simulink model "vipbarcoderecognition"  (R2015b)
settings: Solver=FixedStepDiscrete  StartTime=0.0  StopTime=inf  RelTol=1e-3
undefined symbols (not defined in the file or in its folder): gray, Rec, SDTV
libraries: visiontextngfix x2, simulink x1, visionconversions x1, visionsinks x1, dspvision x1, vipmisc x1
settings Model: FPTRunName=Active  Creator=The MathWorks, Inc.  LastModifiedBy=The MathWorks, Inc.
settings DataIOCC: SaveFormat=Array
settings OptimizationCC: ExpressionDepthLimit=2147483647  EfficientMapNaN2IntZero=off
settings DebuggingCC: UnderspecifiedInitializationDetection=Classic  MergeDetectMultiDrivingBlocksExec=none  SolverPrmCheckMsg=warning  FcnCallInpInsideContextMsg=UseLocalSettings  StateNameClashWarn=warning  StrictBusMsg=Warning
settings HardwareCC: ProdBitPerPointer=32  ProdLargestAtomicFloat=None  ProdIntDivRoundTo=Undefined  ProdEndianess=Unspecified  ProdWordSize=32  ProdHWDeviceType=32-bit Generic  TargetBitPerLong=64  TargetBitPerPointer=64  TargetLongLongMode=on  TargetIntDivRoundTo=Zero  TargetEndianess=LittleEndian  TargetWordSize=64  TargetHWDeviceType=Generic->MATLAB Host Computer  ProdEqTarget=off
settings SFSimCC: SimParseCustomCode=off
settings GRTTargetCC: GeneratePreprocessorConditionals=Disable all  CombineOutputUpdateFcns=off  GRTInterface=on
settings ConfigComp: CovModelRefEnable=Off

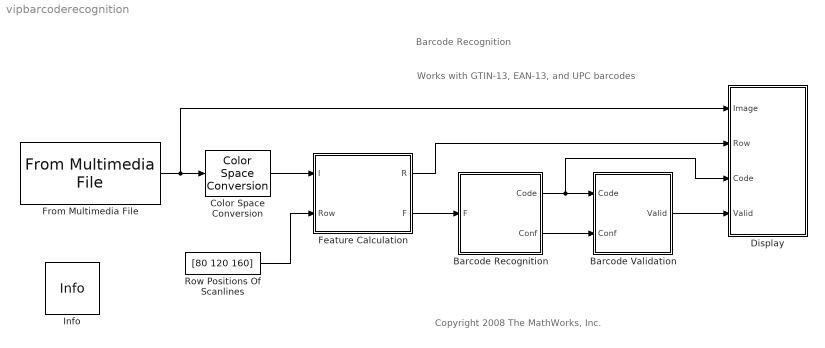
== system vipbarcoderecognition ==
  note: Barcode Recognition
  note: Copyright 2008 The MathWorks, Inc.
  note: Works with GTIN-13, EAN-13, and UPC barcodes
  Barcode Recognition : Subsystem
  Barcode Validation : Subsystem
  Color Space Conversion : visionconversions/Color Space  Conversion  conversion=Obsolete  conversionActive=R'G'B' to intensity  wp_str=D65  rec=Rec. 601 (SDTV)  sys=1125/60/2:1  imagePorts=One multidimensional signal
  Display : Subsystem
  Feature Calculation : MATLAB Function  TreatAsAtomicUnit=on
  From Multimedia File : dspvision/From Multimedia File  inputFilename=vipbarcode.avi  loop=on  numPlays=inf  outputStreams=Video only  videoDataType=single  audioDataType=int16  inheritSampleTime=on  userDefinedSampleTime=1/30  noAudioOutput=off  isIntensityVideo=off  fourcc=RGB  colorVideoFormat=One multidimensional signal  outputEOF=off  dataOrg=Column-major  audioFrameSize=1024  computeAudioFrameSize=off  outSamplingMode=Frame based
  Info : vipmisc/Info  SystemSampleTime=-1
  Row Positions Of Scanlines : Constant  Value=[80 120 160]  VectorParams1D=off  OutDataTypeStr=double
  wires:
  Color Space Conversion/1 -> Feature Calculation/1(I)
  Row Positions Of Scanlines/1 -> Feature Calculation/2(Row)
  From Multimedia File/1 -> Color Space Conversion/1, Display/1(Image)
  Feature Calculation/2(F) -> Barcode Recognition/1(F)
  Barcode Recognition/2(Conf) -> Barcode Validation/2(Conf)
  Barcode Recognition/1(Code) -> Barcode Validation/1(Code), Display/3(Code)
  Barcode Validation/1(Valid) -> Display/4(Valid)
  Feature Calculation/1(R) -> Display/2(Row)

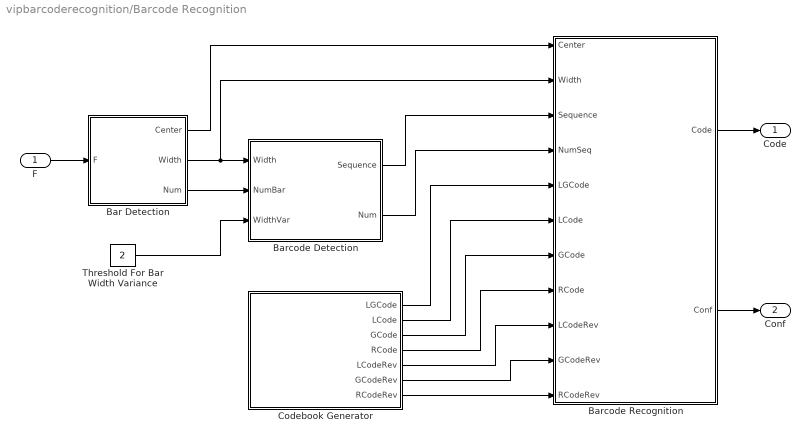
== system vipbarcoderecognition/Barcode Recognition ==
  F : Inport
  Bar Detection : MATLAB Function  TreatAsAtomicUnit=on
  Barcode Detection : MATLAB Function  TreatAsAtomicUnit=on
  Barcode Recognition : MATLAB Function  TreatAsAtomicUnit=on
  Codebook Generator : MATLAB Function  TreatAsAtomicUnit=on
  Threshold For Bar Width Variance : Constant  Value=2  VectorParams1D=off  OutDataTypeStr=single
  Code : Outport
  Conf : Outport  Port=2
  wires:
  Bar Detection/1(Center) -> Barcode Recognition/1(Center)
  Bar Detection/2(Width) -> Barcode Detection/1(Width), Barcode Recognition/2(Width)
  Bar Detection/3(Num) -> Barcode Detection/2(NumBar)
  Barcode Detection/1(Sequence) -> Barcode Recognition/3(Sequence)
  Barcode Detection/2(Num) -> Barcode Recognition/4(NumSeq)
  Codebook Generator/1(LGCode) -> Barcode Recognition/5(LGCode)
  Codebook Generator/2(LCode) -> Barcode Recognition/6(LCode)
  Codebook Generator/3(GCode) -> Barcode Recognition/7(GCode)
  Codebook Generator/4(RCode) -> Barcode Recognition/8(RCode)
  Codebook Generator/7(RCodeRev) -> Barcode Recognition/11(RCodeRev)
  Codebook Generator/5(LCodeRev) -> Barcode Recognition/9(LCodeRev)
  Codebook Generator/6(GCodeRev) -> Barcode Recognition/10(GCodeRev)
  Threshold For Bar Width Variance/1 -> Barcode Detection/3(WidthVar)
  Barcode Recognition/1(Code) -> Code/1
  F/1 -> Bar Detection/1(F)
  Barcode Recognition/2(Conf) -> Conf/1

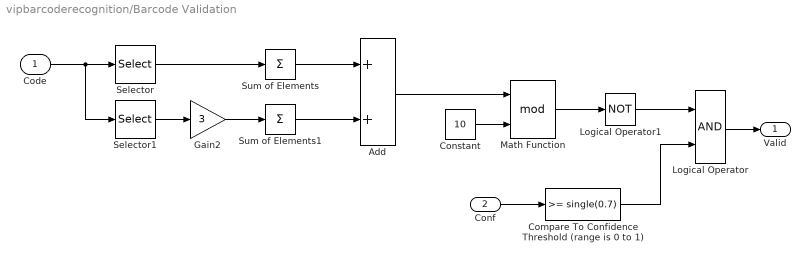
== system vipbarcoderecognition/Barcode Validation ==
  Code : Inport
  Conf : Inport  Port=2
  Add : Sum  AccumDataTypeStr=int32
      settings: AttributesFormatString=Computes\nthe checksum
  Compare To Confidence Threshold (range is 0 to 1) : simulink/Logic and Bit Operations/Compare To Constant  relop=>=  const=single(0.7)  OutDataTypeStr=boolean  ZeroCross=off
  Constant : Constant  Value=10  OutDataTypeStr=int32
  Gain2 : Gain  Gain=3  OutDataTypeStr=Inherit: Inherit via back propagation  ParamDataTypeStr=Inherit: Same as input
  Logical Operator : Logic  AllPortsSameDT=off  OutDataTypeStr=boolean
  Logical Operator1 : Logic  Operator=NOT  AllPortsSameDT=off  OutDataTypeStr=boolean
  Math Function : Math  Operator=mod  SaturateOnIntegerOverflow=on
  Selector : Selector  IndexMode=Zero-based  InputPortWidth=13  IndexOptions=Index vector (dialog)  Indices=[0 2 4 6 8 10 12]  OutputSizes=1
  Selector1 : Selector  IndexMode=Zero-based  InputPortWidth=13  IndexOptions=Index vector (dialog)  Indices=[1 3 5 7 9 11]  OutputSizes=1
  Sum of Elements : Sum  Inputs=+
  Sum of Elements1 : Sum  Inputs=+
  Valid : Outport
  wires:
  Compare To Confidence Threshold (range is 0 to 1)/1 -> Logical Operator/2
  Selector/1 -> Sum of Elements/1
  Selector1/1 -> Gain2/1
  Gain2/1 -> Sum of Elements1/1
  Sum of Elements/1 -> Add/1
  Sum of Elements1/1 -> Add/2
  Add/1 -> Math Function/1
  Code/1 -> Selector/1, Selector1/1
  Logical Operator/1 -> Valid/1
  Conf/1 -> Compare To Confidence Threshold (range is 0 to 1)/1
  Constant/1 -> Math Function/2
  Math Function/1 -> Logical Operator1/1
  Logical Operator1/1 -> Logical Operator/1

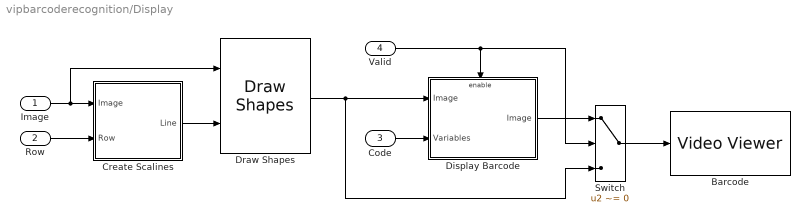
== system vipbarcoderecognition/Display ==
  Image : Inport
  Row : Inport  Port=2
  Code : Inport  Port=3
  Valid : Inport  Port=4
  Barcode : visionsinks/Video Viewer  inputType=Obsolete7b  imagePorts=One multidimensional signal  useColorMap=off  colormapValue=gray(256)  specRange=off  minInputVal=0  maxInputVal=255  FigPos=[290 484 320 262]  AxisZoom=on  trueSizedOnce=on  OpenAtMdlStart=on  DefaultConfigurationName=vipscopes.VideoViewerScopeCfg
  Create Scalines : Subsystem
  Display Barcode : Subsystem  TreatAsAtomicUnit=on
  Draw Shapes : visiontextngfix/Draw Shapes  shape=Lines  fill=off  lineWidth=1  fillClrSource=Specify via dialog  display=User-specified value  intensity=200  color=[1 0 0]  opacity=0.6  viewport=Entire image  antialiasing=off  inType=Obsolete  imagePorts=One multidimensional signal  prodOutputMode=Binary point scaling  prodOutputWordLength=32  prodOutputFracLength=14  memoryMode=Specify word length  memoryWordLength=16  memoryFracLength=15  roundingMode=Floor  overflowMode=off
  Switch : Switch  Criteria=u2 ~= 0
  wires:
  Draw Shapes/1 -> Display Barcode/1(Image), Switch/3
  Switch/1 -> Barcode/1
  Image/1 -> Create Scalines/1(Image), Draw Shapes/1
  Display Barcode/1("Image ") -> Switch/1
  Valid/1 -> Switch/2, Display Barcode/Enable
  Row/1 -> Create Scalines/2(Row)
  Code/1 -> Display Barcode/2(Variables)
  Create Scalines/1(Line) -> Draw Shapes/2

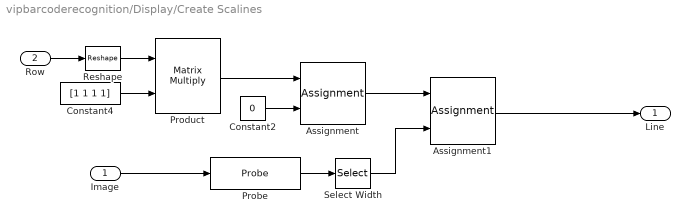
== system vipbarcoderecognition/Display/Create Scalines ==
  Image : Inport
  Row : Inport  Port=2
  Assignment : Assignment  NumberOfDimensions=2  IndexOptions=Assign all,Index vector (dialog)  Indices=1,1  OutputSizes=1,1
  Assignment1 : Assignment  NumberOfDimensions=2  IndexOptions=Assign all,Index vector (dialog)  Indices=3,3  OutputSizes=1,1
  Constant2 : Constant  Value=0  VectorParams1D=off  OutDataTypeStr=Inherit: Inherit via back propagation
  Constant4 : Constant  Value=[1 1 1 1]  VectorParams1D=off  OutDataTypeStr=Inherit: Inherit via back propagation
  Probe : Probe  ProbeWidth=off  ProbeSampleTime=off  ProbeComplexSignal=off  ProbeSignalDimensions=on  ProbeDimensionsDataType=int32
  Product : Product  Multiplication=Matrix(*)  OutDataTypeStr=Inherit: Inherit via back propagation  RndMeth=Zero
  Reshape : Reshape  OutputDimensionality=Column vector (2-D)
  Select Width : Selector  InputPortWidth=3  IndexOptions=Index vector (dialog)  Indices=2  OutputSizes=1
  Line : Outport
  wires:
  Reshape/1 -> Product/1
  Constant4/1 -> Product/2
  Product/1 -> Assignment/1
  Assignment/1 -> Assignment1/1
  Constant2/1 -> Assignment/2
  Probe/1 -> Select Width/1
  Select Width/1 -> Assignment1/2
  Row/1 -> Reshape/1
  Image/1 -> Probe/1
  Assignment1/1 -> Line/1

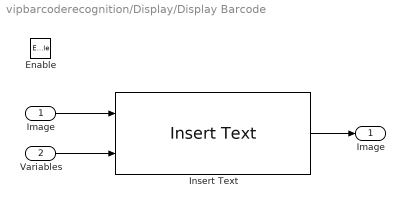
== system vipbarcoderecognition/Display/Display Barcode ==
  Image : Inport
  Variables : Inport  Port=2
  Enable : EnablePort  PropagateVarSize=During execution
  Insert Text : visiontextngfix/Insert Text  inputType=Obsolete  theText='%d%d%d%d%d%d%d%d%d%d%d%d%d'  getTextLocFrom=Specify via dialog  textLoc=[20 20]  getTextColorFrom=Specify via dialog  textColor=[1 1 0]  getTextIntensityFrom=Specify via dialog  textIntensity=0  getTextOpacityFrom=Specify via dialog  textOpacity=1.0  dummyVar2=0  dummyVar3=0  dummyVar4=0  imagePorts=One multidimensional signal  isInputTransposed=off  fontFace=LucidaSansRegular  dummyVar1=0  blockFontSize=28  antiAliased=on
  "Image " : Outport
  wires:
  Image/1 -> Insert Text/1
  Variables/1 -> Insert Text/2
  Insert Text/1 -> "Image "/1

== matlab function vipbarcoderecognition/Barcode Recognition/Codebook Generator ==
  settings: updateMethod=DISCRETE  sampleTime=inf
  data: LGCode output; LCode output; GCode output; RCode output; LCodeRev output; GCodeRev output; RCodeRev output
function [LGCode, LCode, GCode, RCode, LCodeRev, GCodeRev, RCodeRev] = Codebook
UPSAMPLE_RATE = int32(16); % Parameter
% Function CODEBOOK generats the codebooks for GTIN-13.

%--------------------------------------------------------------------------
% Codebook for the first digit which is encoded in the L/G patterns.
%--------------------------------------------------------------------------
ean_code_sym = [ ...
    'LLLLLL'; ... 
    'LLGLGG'; ...
    'LLGGLG'; ...
    'LLGGGL'; ...
    'LGLLGG'; ...
    'LGGLLG'; ...
    'LGGGLL'; ...
    'LGLGLG'; ...
    'LGLGGL'; ...
    'LGGLGL' ];

LGCode = zeros([10, 6], 'int32');
for iNum = 1: 10
    for iSym = 1: 6
        if ean_code_sym(iNum, iSym) == 'L'
            LGCode(iNum, iSym) = iSym;
        else
            LGCode(iNum, iSym) = iSym + 6;
        end
    end
end

%--------------------------------------------------------------------------
% Codebook for the other 12 digits
%--------------------------------------------------------------------------
lcode_sym = [ ...
    '0001101'; ...
    '0011001'; ...
    '0010011'; ...
    '0111101'; ...
    '0100011'; ...
    '0110001'; ...
    '0101111'; ...
    '0111011'; ...
    '0110111'; ...
    '0001011' ];

gcode_sym = [ ...
    '0100111'; ...
    '0110011'; ...
    '0011011'; ...
    '0100001'; ...
    '0011101'; ...
    '0111001'; ...
    '0000101'; ...
    '0010001'; ...
    '0001001'; ...
    '0010111' ];

rcode_sym = [ ...
    '1110010'; ...
    '1100110'; ...
    '1101100'; ...
    '1000010'; ...
    '1011100'; ...
    '1001110'; ...
    '1010000'; ...
    '1000100'; ...
    '1001000'; ...
    '1110100' ];

[LCode] = convertAndUpsample(lcode_sym, UPSAMPLE_RATE);
[GCode] = convertAndUpsample(gcode_sym, UPSAMPLE_RATE);
[RCode] = convertAndUpsample(rcode_sym, UPSAMPLE_RATE);

[LCodeRev] = reverseCodebook(LCode);
[GCodeRev] = reverseCodebook(GCode);
[RCodeRev] = reverseCodebook(RCode);

end

%%%%%%%%%%%%%%%%%%%%%%%%%%%%%%%%%%%%%%%%%%%%%%%%%%%%%%%%%%%%%%%%%%%%%%%%%%%
% Convert the codebook from symbols to digits and upsample them.
%%%%%%%%%%%%%%%%%%%%%%%%%%%%%%%%%%%%%%%%%%%%%%%%%%%%%%%%%%%%%%%%%%%%%%%%%%%
function [codeExpand] = convertAndUpsample(code_sym, UPSAMPLE_RATE)

numCode = size(code_sym, 1);
lenCode = size(code_sym, 2);
codeExpand = zeros([numCode, lenCode*UPSAMPLE_RATE], 'int32');

for iCode = 1: numCode
    for bit = 1: lenCode
        if code_sym(iCode, bit) == '0'
            val = int32(-1);
        else
            val = int32(1);
        end
        
        for idx = (bit-1)*UPSAMPLE_RATE+1: bit*UPSAMPLE_RATE
            codeExpand(iCode, idx) = val;
        end
    end
end
end

%%%%%%%%%%%%%%%%%%%%%%%%%%%%%%%%%%%%%%%%%%%%%%%%%%%%%%%%%%%%%%%%%%%%%%%%%%%
% Reverse the codebook
%%%%%%%%%%%%%%%%%%%%%%%%%%%%%%%%%%%%%%%%%%%%%%%%%%%%%%%%%%%%%%%%%%%%%%%%%%%
function [codeRev] = reverseCodebook(code)
codeRev = code;
lenCode = size(code, 2);
for idx = 1: lenCode
    codeRev(:, idx) = code(:, lenCode-idx+1);
end
end

== matlab function vipbarcoderecognition/Feature Calculation ==
  data: R output; I input; F output; Row input
function [R, F] = Feature(I, Row)
% This function transforms pixels in a given row into a feature vector.

RATIO_STD = single(0.4); % Parameter

% h is a Gaussian filter. It is used to smooth the image gradient which
% indentifies barcode region.
h = single([0.022191, 0.045589, 0.079811, 0.119065, 0.151361, 0.163967, ...
            0.151361, 0.119065, 0.079811, 0.045589, 0.022191]);

% Make sure all scanlines are in valid range.
R = Row;
numRow = size(I, 1);
for idx = 1: numel(R)
    if R(idx) < 1
        R(idx) = 1;
    elseif R(idx) >= numRow
        R(idx) = numRow;
    end
end

F = single(I(R, :));
len = numel(F);

% gradient of the scanlines
gradient = zeros(size(F), 'single');
gradient(2:end-1) = abs(F(3:end) - F(1:end-2));
gradient = conv2(gradient, h, 'same');

% mask consists of most pixels in the barcode region.
mask = (gradient > mean(mean(gradient)));
numPix = single(sum(sum(mask)));
f_mean = single(sum(sum(F .* mask))) / numPix;

% Calculate the mean value and standard deviation for the pixels in the 
% barcode region.
f_std = zeros(1, 'single');
for idx = 1: len
    if mask(idx)
        dif = F(idx) - f_mean;
        f_std = f_std + dif * dif;
    end
end
f_std = sqrt(f_std / numPix);

% Estimate the range of pixel intensity values in the barcode region.
% Values larger than f_high and values smaller than f_low will be saturated.
f_high = f_mean + f_std * RATIO_STD;
f_low  = f_mean - f_std * RATIO_STD;

% Calculate the feature for all pixels in the scanlines. A pixel is 
% classified as black if its value is f_low or less. Black pixels are set
% to 1. A pixel is classified as white if its value is f_high or larger.
% White pixels are set to -1. The remaining pixels are proportionally set 
% to values between -1 and 1.
scale = single(2) / (f_high - f_low);
for iPix = 1: len
    if F(iPix) > f_low && F(iPix) < f_high
        F(iPix) = (f_high - F(iPix)) * scale - single(1);
    elseif F(iPix) <= f_low
        F(iPix) = single(1);
    else
        F(iPix) = single(-1);
    end
end

% Conver the coordinates of from 1-based to 0-based.
R = R - 1;

== matlab function vipbarcoderecognition/Barcode Recognition/Barcode Recognition ==
  data: Center input; Width input; Sequence input; NumSeq input; LGCode input; LCode input; GCode input; RCode input; LCodeRev input; GCodeRev input; RCodeRev input; Code output; Conf output
function [Code, Conf] = Recognition(Center, Width, ...
    Sequence, NumSeq, LGCode, LCode, GCode, RCode, ...
    LCodeRev, GCodeRev, RCodeRev) 
% Function RECOGNITION recognizes the barcode.

% Parameters
UPSAMPLE_RATE = int32(16);

% Constant values
% MID_MODULE is the distance between the first '101' pattern and the middle
% '101' pattern.
MID_MODULE  = int32(46); 
% LAST_MODULE is the distance between the first '101' pattern and the last
% '101' pattern.
LAST_MODULE = int32(92);
% numBinInSym is the number of bins in a symbol
numBinInSym = int32(7 * UPSAMPLE_RATE);

numScanline = numel(NumSeq);
maxNumBar = size(Center, 1);
mapCenter = single(zeros(1, maxNumBar));
mapWidth = single(zeros(1, maxNumBar));
barBin = zeros([1, LAST_MODULE*UPSAMPLE_RATE], 'int32');
    
% Recognize the strings
bestConf = int32(0);
bestCode = zeros([13, 1], 'int32');
codeAll = zeros([13, 1], 'int32');

Center = Center / single(LAST_MODULE);
Width = Width / single(LAST_MODULE);
expCenter = single([0; MID_MODULE; LAST_MODULE]);

for iScanline = 1: numScanline
    for iSequence = 0: NumSeq(iScanline)-1
        dataMx = zeros([3, 3], 'single');
        for iSep = 1: 3
            iBar = Sequence(3*iSequence+iSep, iScanline);
            %loc = mean(bar(1, startBar: startBar+2));
            avgCenter = (Center(iBar, iScanline) ...
                + Center(iBar+1, iScanline) ...
                + Center(iBar+2, iScanline)) / single(3);
            dataMx(iSep, :) = [avgCenter^2, avgCenter, 1];
        end

        coeff = inv(dataMx) * expCenter;

        for iBar = Sequence(3*iSequence+1, iScanline) + 3 ...
                 : Sequence(3*iSequence+3, iScanline) - 1
            mapCenter(iBar) = coeff' * ...
                [Center(iBar, iScanline)^2; Center(iBar, iScanline); 1];
            mapWidth(iBar)  = coeff(1:2)' ...
                * [2*Width(iBar, iScanline); 1] * Width(iBar, iScanline);
        end

        val = int32(-1);
        for iBar = Sequence(3*iSequence+1, iScanline) + 3 ...
                 : Sequence(3*iSequence+3, iScanline) - 1
            left = (mapCenter(iBar) - mapWidth(iBar) / 2) ...
                   * single(UPSAMPLE_RATE);
            right = left + mapWidth(iBar) * single(UPSAMPLE_RATE);
            left = max(left, 1);
            right = min(right, single(LAST_MODULE*UPSAMPLE_RATE));
            for idx = round(left): round(right)
                barBin(idx) = val;
            end
            val = -val;
        end

        leftBin = int32(round(1.5 * UPSAMPLE_RATE));
        rightBin = int32(round(48.5 * UPSAMPLE_RATE));
        
        % Assuming left to right scanline order, recognize digits
        % 8 to 13.
        [rcodeFwd, rconfFwd] = RecognizeHalfCode(RCode, barBin, ...
            rightBin, numBinInSym, false);

        % Assuming right to left scanline order, recognize digits
        % 8 to 13.
        [rcodeRev, rconfRev] = RecognizeHalfCode(RCodeRev, ...
            barBin, leftBin, numBinInSym, true);
        
        % Use the scanline direction (left to right or right to left),
        % find out the potential match for digits 2 to 7.
        if sum(rconfFwd) > sum(rconfRev)
            [lcodeRec, lconfRec] = RecognizeHalfCode(LCode, barBin, ...
                leftBin, numBinInSym, false);
            [gcodeRec, gconfRec] = RecognizeHalfCode(GCode, barBin, ...
                leftBin, numBinInSym, false);
            codeAll(8:13) = rcodeFwd;
            confAll = int32(sum(rconfFwd));
        else
            [lcodeRec, lconfRec] = RecognizeHalfCode(LCodeRev, barBin, ...
                rightBin, numBinInSym, true);
            [gcodeRec, gconfRec] = RecognizeHalfCode(GCodeRev, barBin, ...
                rightBin, numBinInSym, true);
            codeAll(8:13) = rcodeRev;
            confAll = int32(sum(rconfRev));
        end
        
        % Recognize digits 1 to 7.
        [codeLeft, confLeft] = RecognizeFirstHalfCode(LGCode, ...
            lcodeRec, lconfRec, gcodeRec, gconfRec);
        codeAll(1:7) = codeLeft;
        confAll = confAll + confLeft(1);

        if bestConf < confAll
            bestCode = codeAll;
            bestConf = confAll;
        end
    end
end

% Normalize the confidence to [0 1].
Conf = single(bestConf) / single(12*7*UPSAMPLE_RATE);
Code = bestCode;
end



%%%%%%%%%%%%%%%%%%%%%%%%%%%%%%%%%%%%%%%%%%%%%%%%%%%%%%%%%%%%%%%%%%%%%%%%%%%
% Recognize the first 7 digits
%%%%%%%%%%%%%%%%%%%%%%%%%%%%%%%%%%%%%%%%%%%%%%%%%%%%%%%%%%%%%%%%%%%%%%%%%%%
function [code, conf] = ...
    RecognizeFirstHalfCode(LGCode, lcode, lconf, gcode, gconf)
codeComb = [lcode, gcode];
confComb = [lconf, gconf];
code = zeros([7, 1], 'int32');
conf = zeros([7, 1], 'int32');

bestCode = 1;
bestSum = sum(confComb(LGCode(bestCode, :)));
for idx = 2: 10
    curSum = sum(confComb(LGCode(idx, :)));
    if bestSum < curSum
        bestCode = idx;
        bestSum = curSum;
    end
end

code(1) = bestCode - int32(1);
conf(1) = bestSum;
code(2:7) = codeComb(LGCode(bestCode, :));
conf(2:7) = confComb(LGCode(bestCode, :));
end

%%%%%%%%%%%%%%%%%%%%%%%%%%%%%%%%%%%%%%%%%%%%%%%%%%%%%%%%%%%%%%%%%%%%%%%%%%%
% Recognize half of the barcode by comparing them with a codebook
%%%%%%%%%%%%%%%%%%%%%%%%%%%%%%%%%%%%%%%%%%%%%%%%%%%%%%%%%%%%%%%%%%%%%%%%%%%
function [code, conf] = RecognizeHalfCode(codebook, barBin, ...
    firstBin, numBinInSym, isReverse)
code = zeros([6, 1], 'int32');
conf = zeros([6, 1], 'int32');

iSym = 1;
step = 1;
if isReverse
    iSym = 6;
    step = -1;
end

startBin = firstBin;
for idx = 1: 6
    bestCode = int32(0);
    bestSum = -2*numBinInSym;
    for iCode = int32(1): int32(10)
        sum = int32(0);
        for jdx = 1: numBinInSym
            sum = sum + barBin(startBin+jdx-1) * codebook(iCode, jdx);
        end
        
        if bestSum < sum
            bestSum = sum;
            bestCode = iCode;
        end
    end
    code(iSym) = bestCode - int32(1);
    conf(iSym) = bestSum;
    iSym = iSym + step;
    startBin = startBin + numBinInSym;
end
end

== matlab function vipbarcoderecognition/Barcode Recognition/Bar Detection ==
  data: F input; Center output; Width output; Num output
function [Center, Width, Num] = Bar(F)
% Function BAR detects bars from barcode feature signal.

MAX_BAR_NUM = 200;
[numFeature, lenFeature] = size(F);
Center = zeros([MAX_BAR_NUM, numFeature], 'single');
Width = zeros([MAX_BAR_NUM, numFeature], 'single');
Num = zeros([1, numFeature], 'int32');

for iFeature = 1: numFeature
    iBar = 0;
    iPix = 1;
    
    % First, try to find a black bar.
    % If it is not there, the first bar has zero width.
    while iPix <= lenFeature && iBar < MAX_BAR_NUM
        % Find a black bar.
        % A contiguous sequence of pixels with zero or positive feature
        % value is considered a black bar.
        curWidth  = zeros(1, 'single');
        curCenter = zeros(1, 'single');
        while iPix <= lenFeature && F(iFeature, iPix) >= 0
            curWidth  = curWidth + F(iFeature, iPix);
            curCenter = curCenter + F(iFeature, iPix) * iPix;
            iPix = iPix + 1;
        end

        iBar = iBar + 1;
        if curWidth > 0
            Center(iBar, iFeature) = curCenter / curWidth;
            Width(iBar, iFeature) = curWidth;
        end

        % Find a white bar.
        % A contiguous sequence of pixels with negative feature
        % value is considered a white bar.
        curWidth  = zeros(1, 'single');
        curCenter = zeros(1, 'single');
        while iPix <= lenFeature && F(iFeature, iPix) < 0
            curWidth  = curWidth + F(iFeature, iPix);
            curCenter = curCenter + F(iFeature, iPix) * iPix;
            iPix = iPix + 1;
        end

        if curWidth < 0 && iBar < MAX_BAR_NUM
            iBar = iBar + 1;
            Center(iBar, iFeature) = curCenter / curWidth;
            Width(iBar, iFeature) = -curWidth;
        end
    end
    Num(1, iFeature) = iBar;
end

== matlab function vipbarcoderecognition/Barcode Recognition/Barcode Detection ==
  data: Width input; NumBar input; Sequence output; Num output; WidthVar input
function [Sequence, Num] = Detection(Width, NumBar, WidthVar)
% DETECTION returns sequence of indices to barcode guard bars

% Parameters
WIDTH_VAR_DETECT = WidthVar;
BAR_VAR_NUM = 1;

% Maximum signal dimensions
MAX_SEP_NUM = 50; % max number of guard patterns (separators)
MAX_SEQ_NUM = 30; % max number of sequences of guard patterns

% Constant values
BAR_END2END_NUM = 56; % count of both black and white bars
BAR_END2MID_NUM = 28;

numScanline = numel(NumBar);
separator = zeros([1, MAX_SEP_NUM], 'int32');
Sequence = zeros([3*MAX_SEQ_NUM, numScanline], 'int32');
Num = zeros([1, numScanline], 'int32');

for iScanline = 1: numScanline
    % Calculate sequence and its length
    firstBar = 1;
    % Skip the first bar if it's invalid
    if Width(firstBar) == 0
        firstBar = firstBar + 2;
    end

    % Find out all possible separators
    numSep = 0;
    while firstBar <= NumBar(iScanline)-2
        [avgWidth, devWidth] = Statistics(Width, iScanline, firstBar, 3);
        if numSep < MAX_SEP_NUM && devWidth < WIDTH_VAR_DETECT; % * dis_mean
            numSep = numSep + 1;
            separator(numSep) = firstBar;
        end
        firstBar = firstBar + 2;
    end

    % Find out sequences of bars that may form a valid barcode string
    iSequence = 0;
    iStart = 1;
    lastStartSep = NumBar(iScanline) - BAR_END2END_NUM + 2 * BAR_VAR_NUM;
    while iSequence < MAX_SEQ_NUM ...
            && iStart <= numSep-2 && separator(iStart) <= lastStartSep
        firstMidSep = separator(iStart) + BAR_END2MID_NUM - 2 * BAR_VAR_NUM;
        lastMidSep  = firstMidSep + 4 * BAR_VAR_NUM;
        firstEndSep = separator(iStart) + BAR_END2END_NUM - 2 * BAR_VAR_NUM;
        lastEndSep  = firstEndSep + 4 * BAR_VAR_NUM;
        
        % Skip the first part
        iMid = iStart + 1;
        while iMid <= numSep-1 && separator(iMid) < firstMidSep
            iMid = iMid + 1;
        end

        while iSequence < MAX_SEQ_NUM ...
                && iMid <= numSep-1 && separator(iMid) <= lastMidSep
            % Skip the first part
            iEnd = iMid + 1;
            while iEnd <= numSep && separator(iEnd) < firstEndSep
                iEnd = iEnd + 1;
            end

            while iSequence < MAX_SEQ_NUM ...
                    && iEnd <= numSep && separator(iEnd) <= lastEndSep
                avgWidth = zeros(1, 'single');
                for iBar = separator(iStart): separator(iStart)+2
                    avgWidth = avgWidth + Width(iBar, iScanline);
                end
                for iBar = separator(iEnd): separator(iEnd)+2
                    avgWidth = avgWidth + Width(iBar, iScanline);
                end
                avgWidth = avgWidth / single(6);

                devWidth = zeros(1, 'single');
                for iBar = separator(iMid)-1: separator(iMid)+3
                    difWidth = abs(Width(iBar, iScanline) - avgWidth);
                    if devWidth < difWidth
                        devWidth = difWidth;
                    end
                end

                if devWidth < WIDTH_VAR_DETECT; % * dis_mean_exp
                    Sequence(3*iSequence+1, iScanline) = separator(iStart);
                    Sequence(3*iSequence+2, iScanline) = separator(iMid);
                    Sequence(3*iSequence+3, iScanline) = separator(iEnd);
                    iSequence = iSequence + 1;
                end
                iEnd = iEnd + 1;
            end
            iMid = iMid + 1;
        end

        iStart = iStart + 1;
    end
    Num(iScanline) = iSequence;
end
end

%%%%%%%%%%%%%%%%%%%%%%%%%%%%%%%%%%%%%%%%%%%%%%%%%%%%%%%%%%%%%%%%%%%%%%%%%%%
% Calculate the average and deviation of the data
%%%%%%%%%%%%%%%%%%%%%%%%%%%%%%%%%%%%%%%%%%%%%%%%%%%%%%%%%%%%%%%%%%%%%%%%%%%
function [avg, dev] = Statistics(data, col, first, Num)
avg = zeros(1, 'single');
for idx = first: first+Num-1
    avg = avg + data(idx, col);
end
avg = avg / Num;

dev = zeros(1, 'single');
for idx = first : first+Num-1
    dif = abs(data(idx, col) - avg);
    if dev < dif
        dev = dif;
    end
end
end
